simulink model "lab03fig02"  (R2015a)
settings: Solver=ode45  StartTime=0.0  StopTime=100.0  RelTol=1e-3
settings Model: Creator=dg  LastModifiedBy=dg

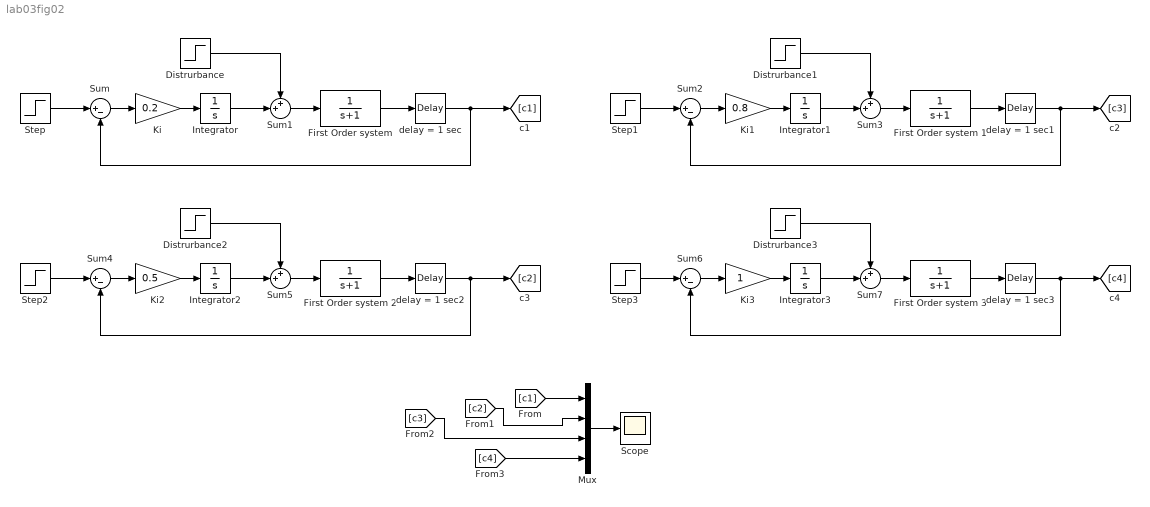
== system lab03fig02 ==
  Distrurbance{,1..3} (4 alike) : Step  Time=25  SampleTime=0
  First Order system {,1..3} (4 alike) : TransferFcn  Denominator=[1 1]
  Integrator{,1..3} (4 alike) : Integrator
  Ki : Gain  Gain=0.2
  Ki1 : Gain  Gain=0.8
  Ki2 : Gain  Gain=0.5
  Ki3 : Gain
  Mux : Mux
  Scope : Scope
  Step{,1..3} (4 alike) : Step  SampleTime=0
  Sum{,2,4,6} (4 alike) : Sum  Inputs=|+-
  Sum{1,3,5,7} (4 alike) : Sum  Inputs=++|
  delay = 1 sec{,1..3} (4 alike) : TransportDelay
  wires:
  Distrurbance/1 -> Sum1/1
  Step/1 -> Sum/1
  Sum/1 -> Ki/1
  Ki/1 -> Integrator/1
  Integrator/1 -> Sum1/2
  Sum1/1 -> "First Order system "/1
  "First Order system "/1 -> delay = 1 sec/1
  delay = 1 sec/1 -> [c1], Sum/2
  [c1] -> Mux/1
  Distrurbance1/1 -> Sum3/1
  Step1/1 -> Sum2/1
  Sum2/1 -> Ki1/1
  Ki1/1 -> Integrator1/1
  Integrator1/1 -> Sum3/2
  Sum3/1 -> First Order system 1/1
  First Order system 1/1 -> delay = 1 sec1/1
  delay = 1 sec1/1 -> [c3], Sum2/2
  Distrurbance2/1 -> Sum5/1
  Step2/1 -> Sum4/1
  Sum4/1 -> Ki2/1
  Ki2/1 -> Integrator2/1
  Integrator2/1 -> Sum5/2
  Sum5/1 -> First Order system 2/1
  First Order system 2/1 -> delay = 1 sec2/1
  delay = 1 sec2/1 -> [c2], Sum4/2
  Distrurbance3/1 -> Sum7/1
  Step3/1 -> Sum6/1
  Sum6/1 -> Ki3/1
  Ki3/1 -> Integrator3/1
  Integrator3/1 -> Sum7/2
  Sum7/1 -> First Order system 3/1
  First Order system 3/1 -> delay = 1 sec3/1
  delay = 1 sec3/1 -> [c4], Sum6/2
  [c2] -> Mux/2
  [c3] -> Mux/3
  [c4] -> Mux/4
  Mux/1 -> Scope/1
